simulink model "SuspensionCar"  (R2021a)
settings: Solver=VariableStepAuto  StartTime=0.0  StopTime=70  RelTol=1e-3
values from neighbouring files (symbols this model uses):
  b1 = 350    [Parameter.m]
  b2 = 15020    [Parameter.m]
  k1 = 80000    [Parameter.m]
  k2 = 500000    [Parameter.m]
  m1 = 2500    [Parameter.m]
  m2 = 320    [Parameter.m]
libraries: fuzblock x1, slpidlib x1
settings Model: Creator=Azriel  LastModifiedBy=Azriel

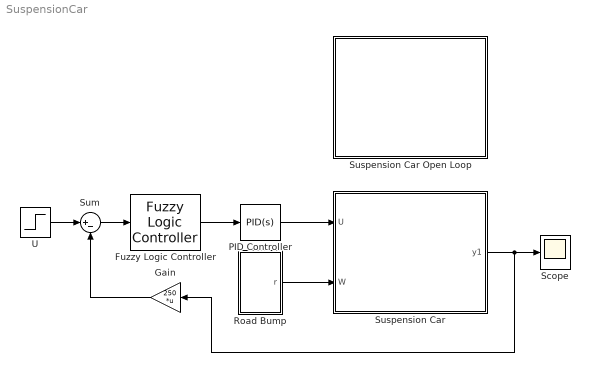
== system SuspensionCar ==
  Fuzzy Logic Controller : fuzblock/Fuzzy Logic  Controller  FIS='Sus.fis'  OutputSampleNumber=101  DataType=double  FuzzifiedInputs=off  RuleFiringStrengths=off  RuleOutputs=off  AggregatedOutputs=off  SimulateUsing=Interpreted execution  OutOfRangeInputValueMessage=warning  NoRuleFiredMessage=warning  EmptyOutputFuzzySetMessage=warning
  Gain : Gain  Gain=250  Multiplication=Matrix(K*u)
  PID Controller : slpidlib/PID Controller  Controller=PID  Form=Parallel  TimeDomain=Continuous-time  UseExternalTs=off  SampleTime=-1  IntegratorMethod=Forward Euler  FilterMethod=Forward Euler  ControllerParametersSource=internal  P=10  I=5  D=1  UseFilter=on  N=100  TunerSelectOption=Transfer Function Based (PID Tuner App)  InitialConditionSource=internal  InitialConditionForIntegrator=0  InitialConditionForFilter=0  DifferentiatorICPrevScaledInput=0  ExternalReset=none  TrackingMode=off  Kt=1  LimitOutput=off  SatLimitsSource=internal  UpperSaturationLimit=inf  LowerSaturationLimit=-inf  LinearizeAsGain=on  AntiWindupMode=none  Kb=1  POutMin=[]  POutMax=[]  IOutMin=[]  IOutMax=[]  DOutMin=[]  DOutMax=[]  NOutMin=[]  NOutMax=[]  SumOutMin=[]  SumOutMax=[]  SaturationOutMin=[]  SaturationOutMax=[]  PParamMin=[]  PParamMax=[]  IParamMin=[]  IParamMax=[]  DParamMin=[]  DParamMax=[]  NParamMin=[]  NParamMax=[]  KbParamMin=[]  KbParamMax=[]  KtParamMin=[]  KtParamMax=[]  KbOutMin=[]  KbOutMax=[]  KtOutMin=[]  KtOutMax=[]  IntegratorOutMin=[]  IntegratorOutMax=[]  FilterOutMin=[]  FilterOutMax=[]  SumI1OutMin=[]  SumI1OutMax=[]  SumI2OutMin=[]  SumI2OutMax=[]  SumI3OutMin=[]  SumI3OutMax=[]  SumI4OutMin=[]  SumI4OutMax=[]  SumDOutMin=[]  SumDOutMax=[]  DifferentiatorOutMin=[]  DifferentiatorOutMax=[]  FilterDiffOutCoefMin=[]  FilterDiffOutCoefMax=[]  ReciprocalOutMin=[]  ReciprocalOutMax=[]  SumDenOutMin=[]  SumDenOutMax=[]  SumNumOutMin=[]  SumNumOutMax=[]  DivideOutMin=[]  DivideOutMax=[]  UdiffTsProdOutMin=[]  UdiffTsProdOutMax=[]  NTsProdOutMin=[]  NTsProdOutMax=[]  UintegralTsProdOutMin=[]  UintegralTsProdOutMax=[]  UngainTsProdOutMin=[]  UngainTsProdOutMax=[]  IntegratorContinuousStateAttributes=''  IntegratorStateMustResolveToSignalObject=off  IntegratorRTWStateStorageClass=Auto  FilterContinuousStateAttributes=''  FilterStateMustResolveToSignalObject=off  FilterRTWStateStorageClass=Auto  ParallelPVariant=InternalParameters  IdealPVariant=Disabled  IVariant=InternalParameters  DVariant=InternalParameters  IntegratorVariant=Continuous  SatVariant=Disabled  AWVariant=Passthrough  PCopyVariant=Disabled  TRVariant=Disabled  FdbkBlocksVariant=Forward  IdealPFdbkVariant=Disabled  SatFdbkVariant=Disabled  DerivativeFilterVariant=ContFilter  NVariant=InternalParameters  NCopyVariant=Disabled  FilterICVariant=InternalICsFilter  IntegratorICVariant=InternalICs  ExternalResetVariant=Disabled  TRSumVariant=Passthrough  SumFdbkVariant=Disabled  SumVariant=Sum_PID  TsampFilterVariant=InternalTs  TsampNgainVariant=Passthrough  TsampIntegralVariant=Passthrough  ExternalSaturationOutDataTypeStr=Inherit: Same as second input
  Road Bump : Subsystem
  Scope : Scope
  Sum : Sum  Inputs=|+-
  Suspension Car : Subsystem
  Suspension Car Open Loop : Subsystem
  U : Step  Time=0  After=0  SampleTime=0
  wires:
  Suspension Car/1(y1) -> Scope/1, Gain/1
  Road Bump/1(r) -> Suspension Car/2(W)
  Sum/1 -> Fuzzy Logic Controller/1
  U/1 -> Sum/1
  Gain/1 -> Sum/2
  Fuzzy Logic Controller/1 -> PID Controller/1
  PID Controller/1 -> Suspension Car/1(U)

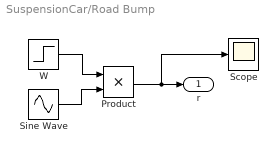
== system SuspensionCar/Road Bump ==
  Product : Product
  Scope : Scope
  Sine Wave : Sin  Amplitude=6  Frequency=0.5  SampleTime=0
  W : Step  Time=0  After=-0.5  SampleTime=0
  r : Outport
  wires:
  Product/1 -> Scope/1, r/1
  W/1 -> Product/1
  Sine Wave/1 -> Product/2

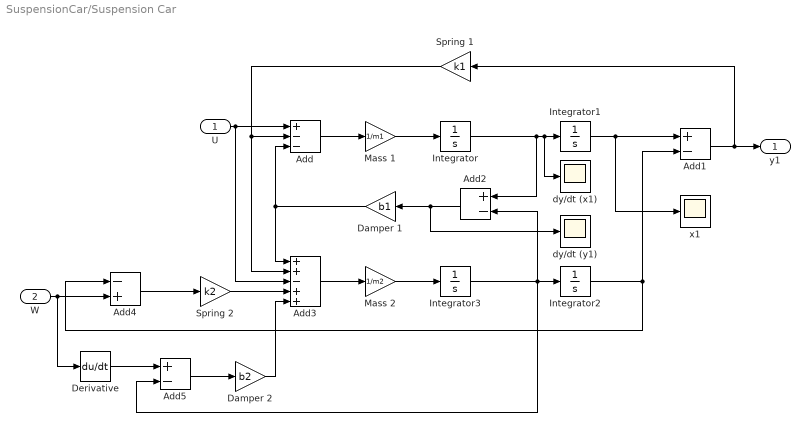
== system SuspensionCar/Suspension Car ==
  U : Inport
  W : Inport  Port=2
  Add : Sum  Inputs=+--
  Add1 : Sum  Inputs=+-
  Add2 : Sum  Inputs=+-
  Add3 : Sum  Inputs=+|+|-|+|+
  Add4 : Sum  Inputs=-+
  Add5 : Sum  Inputs=+-
  Damper 1 : Gain  Gain=b1
  Damper 2 : Gain  Gain=b2
  Derivative : Derivative
  Integrator{,1..3} (4 alike) : Integrator
  Mass 1 : Gain  Gain=1/m1
  Mass 2 : Gain  Gain=1/m2
  Spring 1 : Gain  Gain=k1
  Spring 2 : Gain  Gain=k2
  dy/dt (x1) : Scope
  dy/dt (y1) : Scope
  x1 : Scope
  y1 : Outport
  wires:
  Damper 1/1 -> Add/3, Add3/1
  W/1 -> Add4/2, Derivative/1
  Mass 2/1 -> Integrator3/1
  Add2/1 -> dy/dt (y1)/1, Damper 1/1
  Integrator3/1 -> Integrator2/1, Add2/2, Add5/2
  Add5/1 -> Damper 2/1
  Spring 1/1 -> Add/2, Add3/2
  U/1 -> Add3/3, Add/1
  Integrator/1 -> dy/dt (x1)/1, Integrator1/1, Add2/1
  Mass 1/1 -> Integrator/1
  Integrator1/1 -> x1/1, Add1/1
  Add3/1 -> Mass 2/1
  Integrator2/1 -> Add1/2, Add4/1
  Damper 2/1 -> Add3/5
  Add/1 -> Mass 1/1
  Add1/1 -> y1/1, Spring 1/1
  Spring 2/1 -> Add3/4
  Derivative/1 -> Add5/1
  Add4/1 -> Spring 2/1

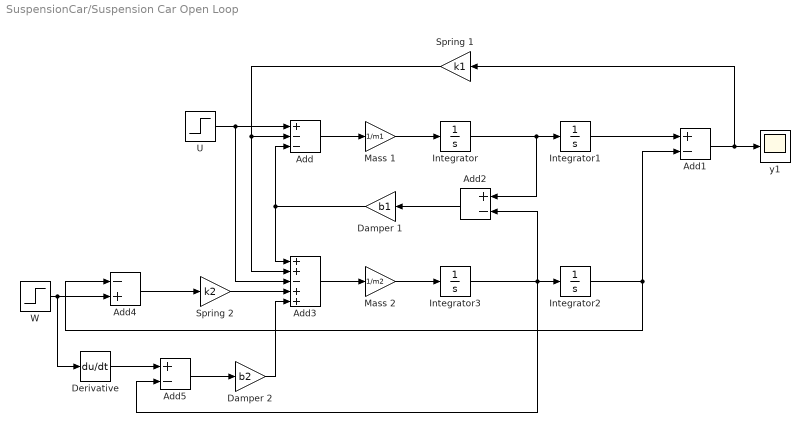
== system SuspensionCar/Suspension Car Open Loop ==
  Add : Sum  Inputs=+--
  Add1 : Sum  Inputs=+-
  Add2 : Sum  Inputs=+-
  Add3 : Sum  Inputs=+|+|-|+|+
  Add4 : Sum  Inputs=-+
  Add5 : Sum  Inputs=+-
  Damper 1 : Gain  Gain=b1
  Damper 2 : Gain  Gain=b2
  Derivative : Derivative
  Integrator{,1..3} (4 alike) : Integrator
  Mass 1 : Gain  Gain=1/m1
  Mass 2 : Gain  Gain=1/m2
  Spring 1 : Gain  Gain=k1
  Spring 2 : Gain  Gain=k2
  U : Step  Time=0  After=0  SampleTime=0
  W : Step  Time=0  After=-0.5  SampleTime=0
  y1 : Scope
  wires:
  Damper 1/1 -> Add/3, Add3/1
  W/1 -> Add4/2, Derivative/1
  Mass 2/1 -> Integrator3/1
  Add2/1 -> Damper 1/1
  Integrator3/1 -> Integrator2/1, Add2/2, Add5/2
  Add5/1 -> Damper 2/1
  Spring 1/1 -> Add/2, Add3/2
  U/1 -> Add3/3, Add/1
  Integrator/1 -> Integrator1/1, Add2/1
  Mass 1/1 -> Integrator/1
  Integrator1/1 -> Add1/1
  Add3/1 -> Mass 2/1
  Integrator2/1 -> Add1/2, Add4/1
  Damper 2/1 -> Add3/5
  Add/1 -> Mass 1/1
  Add1/1 -> y1/1, Spring 1/1
  Spring 2/1 -> Add3/4
  Derivative/1 -> Add5/1
  Add4/1 -> Spring 2/1
